simulink model "holiday4"  (R2019a)
settings: Solver=VariableStepAuto  StartTime=0.0  StopTime=10.0  RelTol=1e-3
settings Model: Creator=Aditya  LastModifiedBy=Aditya

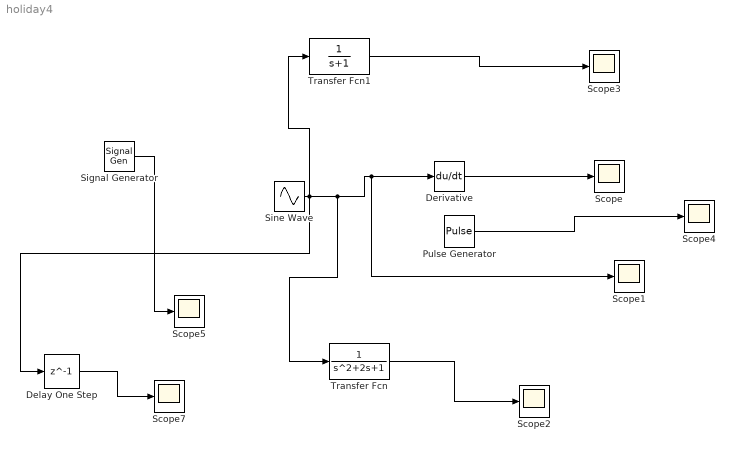
== system holiday4 ==
  Delay One Step : Delay  DelayLength=1
  Derivative : Derivative
  Pulse Generator : DiscretePulseGenerator  PulseType=Time based  Period=10  PulseWidth=5
  Scope{,1..5,7} (7 alike) : Scope
  Signal Generator : SignalGenerator  WaveForm=sawtooth  Units=rad/sec
  Sine Wave : Sin  SampleTime=0
  Transfer Fcn : TransferFcn
  Transfer Fcn1 : TransferFcn  Denominator=[1 1]
  wires:
  Sine Wave/1 -> Delay One Step/1, Transfer Fcn1/1, Transfer Fcn/1, Derivative/1, Scope1/1
  Derivative/1 -> Scope/1
  Transfer Fcn/1 -> Scope2/1
  Transfer Fcn1/1 -> Scope3/1
  Pulse Generator/1 -> Scope4/1
  Signal Generator/1 -> Scope5/1
  Delay One Step/1 -> Scope7/1
